simulink model "msdft_comb"  (R2013b)
settings: Solver=ode45  StartTime=0.0  StopTime=10.0  RelTol=1e-3
libraries: xbsIndex_r4 x10, casper_library_misc x3
settings Model: Creator=root  LastModifiedBy=root

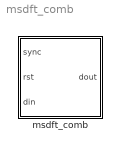
== system msdft_comb ==
  msdft_comb : Subsystem  mask(msdft_comb){input_bitsize=10, fft_len=10, latency=0}
      mask prompts: fft_len "fft_len (2^?)"; latency "sub latency"
      mask init:
      | msdft_comb_init(gcb, ...
      |         'input_bitsize', input_bitsize, ...
      |         'fft_len', fft_len, ...
      |         'latency', latency);
      settings: AttributesFormatString=latency=0

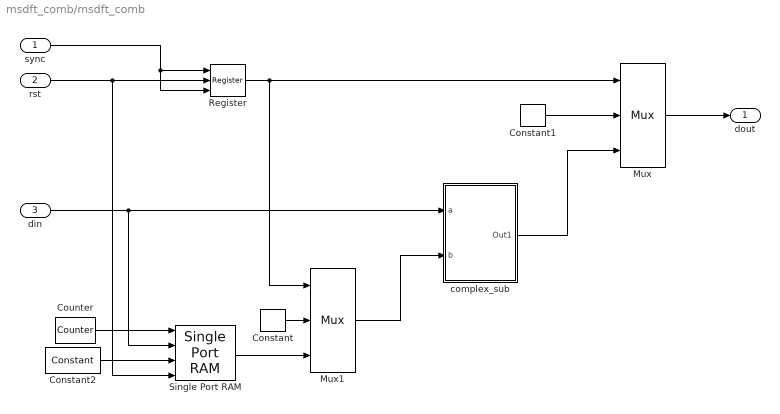
== system msdft_comb/msdft_comb ==
  sync : Inport
  rst : Inport  Port=2
  din : Inport  Port=3
  Constant : xbsIndex_r4/Constant  const=0  gui_display_data_type=Fixed-point  arith_type=Unsigned  n_bits=2*input_bitsize  bin_pt=0  preci_type=Single  exp_width=8  frac_width=24  explicit_period=on  period=1  equ=P=C  opselect=C  inp2=PCIN>>17  opr=+  inp1=P  carry=CIN  dbl_ovrd=off  block_type=constant
  Constant1 : xbsIndex_r4/Constant  const=0  gui_display_data_type=Fixed-point  arith_type=Unsigned  n_bits=2*(input_bitsize+1)  bin_pt=0  preci_type=Single  exp_width=8  frac_width=24  explicit_period=on  period=1  equ=P=C  opselect=C  inp2=PCIN>>17  opr=+  inp1=P  carry=CIN  dbl_ovrd=off  block_type=constant
  Constant2 : xbsIndex_r4/Constant  const=1  gui_display_data_type=Boolean  arith_type=Boolean  n_bits=16  bin_pt=14  preci_type=Single  exp_width=8  frac_width=24  explicit_period=on  period=1  equ=P=C  opselect=C  inp2=PCIN>>17  opr=+  inp1=P  carry=CIN  dbl_ovrd=off  block_type=constant
  Counter : xbsIndex_r4/Counter  cnt_type=Free Running  cnt_to=Inf  operation=Up  start_count=0  cnt_by_val=1  arith_type=Unsigned  n_bits=fft_len  bin_pt=0  load_pin=off  rst=off  en=off  explicit_period=on  period=1  dbl_ovrd=off  use_behavioral_HDL=off  implementation=Fabric  block_type=counter
  Mux : xbsIndex_r4/Mux  inputs=2  en=off  latency=0  precision=Full  arith_type=Unsigned  n_bits=16  bin_pt=14  quantization=Truncate  overflow=Wrap  dbl_ovrd=off  block_type=mux
  Mux1 : xbsIndex_r4/Mux  inputs=2  en=off  latency=0  precision=Full  arith_type=Unsigned  n_bits=16  bin_pt=14  quantization=Truncate  overflow=Wrap  dbl_ovrd=off  block_type=mux
  Register : xbsIndex_r4/Register  init=0  rst=on  en=on  dbl_ovrd=off  block_type=register
  Single Port RAM : xbsIndex_r4/Single Port RAM  depth=2^fft_len  initVector=sin(pi*(0:15)/16)  distributed_mem=Block RAM  write_mode=Read Before Write  rst=on  init_reg=0  en=off  latency=1  dbl_ovrd=off  optimize=Area  block_type=spram
  complex_sub : Subsystem  mask(complex_sub){a_bitsize=input_bitsize, b_bitsize=input_bitsize, latency=0}
      mask init:
      | complex_sub_init(gcb, ...
      |             'a_bitsize', a_bitsize, ...
      |             'b_bitsize', b_bitsize, ...
      |             'latency', latency);
      settings: AttributesFormatString=latency=0
  dout : Outport
  wires:
  sync/1 -> Register/3, Register/1
  rst/1 -> Single Port RAM/4, Register/2
  Register/1 -> Mux1/1, Mux/1
  din/1 -> Single Port RAM/2, complex_sub/1("a ")
  complex_sub/1(Out1) -> Mux/3
  Single Port RAM/1 -> Mux1/3
  Constant/1 -> Mux1/2
  Constant1/1 -> Mux/2
  Mux1/1 -> complex_sub/2(b)
  Mux/1 -> dout/1
  Constant2/1 -> Single Port RAM/3
  Counter/1 -> Single Port RAM/1

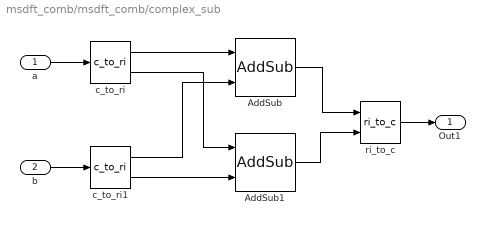
== system msdft_comb/msdft_comb/complex_sub ==
  "a " : Inport
  b : Inport  Port=2
  AddSub : xbsIndex_r4/AddSub  mode=Subtraction  use_carryin=off  use_carryout=off  en=off  latency=latency  precision=Full  arith_type=Unsigned  n_bits=16  bin_pt=14  quantization=Truncate  overflow=Wrap  dbl_ovrd=off  use_behavioral_HDL=off  hw_selection=Fabric  pipelined=off  block_type=addsub
  AddSub1 : xbsIndex_r4/AddSub  mode=Subtraction  use_carryin=off  use_carryout=off  en=off  latency=latency  precision=Full  arith_type=Unsigned  n_bits=16  bin_pt=14  quantization=Truncate  overflow=Wrap  dbl_ovrd=off  use_behavioral_HDL=off  hw_selection=Fabric  pipelined=off  block_type=addsub
  c_to_ri : casper_library_misc/c_to_ri  n_bits=a_bitsize  bin_pt=a_bitsize-1
      settings: AttributesFormatString=10_9 r/i
  c_to_ri1 : casper_library_misc/c_to_ri  n_bits=b_bitsize  bin_pt=b_bitsize-1
      settings: AttributesFormatString=0_-1 r/i
  ri_to_c : casper_library_misc/ri_to_c
  Out1 : Outport
  wires:
  "a "/1 -> c_to_ri/1
  b/1 -> c_to_ri1/1
  c_to_ri/1 -> AddSub/1
  c_to_ri1/1 -> AddSub/2
  c_to_ri/2 -> AddSub1/1
  c_to_ri1/2 -> AddSub1/2
  AddSub/1 -> ri_to_c/1
  AddSub1/1 -> ri_to_c/2
  ri_to_c/1 -> Out1/1
